simulink model "operator2"  (Simulink 8.1)
settings: Solver=ode45  StartTime=0.0  StopTime=inf  RelTol=1e-3
settings Model: Creator=eiseles  LastModifiedBy=eiseles
settings DataIOCC: SignalLoggingSaveFormat=Dataset
settings OptimizationCC: ExpressionDepthLimit=128
settings DebuggingCC: FcnCallInpInsideContextMsg=EnableAllAsError
settings GRTTargetCC: CombineOutputUpdateFcns=on  GRTInterface=off

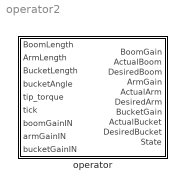
== system operator2 ==
  operator : Subsystem

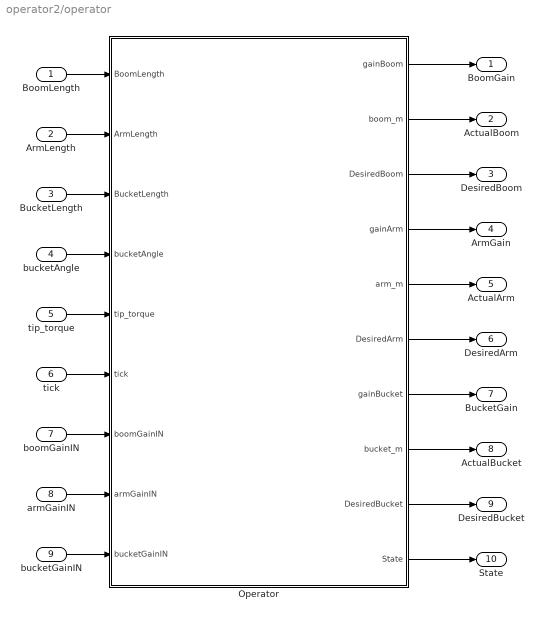
== system operator2/operator ==
  BoomLength : Inport
  ArmLength : Inport  Port=2
  BucketLength : Inport  Port=3
  bucketAngle : Inport  Port=4
  tip_torque : Inport  Port=5
  tick : Inport  Port=6
  boomGainIN : Inport  Port=7
  armGainIN : Inport  Port=8
  bucketGainIN : Inport  Port=9
  Operator : Stateflow chart  TreatAsAtomicUnit=on
  BoomGain : Outport
  ActualBoom : Outport  Port=2
  DesiredBoom : Outport  Port=3
  ArmGain : Outport  Port=4
  ActualArm : Outport  Port=5
  DesiredArm : Outport  Port=6
  BucketGain : Outport  Port=7
  ActualBucket : Outport  Port=8
  DesiredBucket : Outport  Port=9
  State : Outport  Port=10
  wires:
  bucketAngle/1 -> Operator/4(bucketAngle)
  BoomLength/1 -> Operator/1(BoomLength)
  BucketLength/1 -> Operator/3(BucketLength)
  tip_torque/1 -> Operator/5(tip_torque)
  ArmLength/1 -> Operator/2(ArmLength)
  Operator/2(boom_m) -> ActualBoom/1
  Operator/3(DesiredBoom) -> DesiredBoom/1
  Operator/4(gainArm) -> ArmGain/1
  Operator/1(gainBoom) -> BoomGain/1
  Operator/6(DesiredArm) -> DesiredArm/1
  Operator/7(gainBucket) -> BucketGain/1
  Operator/9(DesiredBucket) -> DesiredBucket/1
  Operator/5(arm_m) -> ActualArm/1
  Operator/8(bucket_m) -> ActualBucket/1
  tick/1 -> Operator/6(tick)
  Operator/10(State) -> State/1
  boomGainIN/1 -> Operator/7(boomGainIN)
  armGainIN/1 -> Operator/8(armGainIN)
  bucketGainIN/1 -> Operator/9(bucketGainIN)

== stateflow chart operator/Operator ==
  state captured
    entry: State= 1;
    boom_m = BoomLength;
    arm_m = ArmLength;
    bucket_m = -bucketAngle;
    DesiredBoom = .08;
    DesiredArm = .99;
    DesiredBucket = levelBucket;
    during:boom_m = BoomLength;
    arm_m = ArmLength;
    bucket_m = -bucketAngle;
  state Lifting
    entry: State= 2;
    boom_m = BoomLength;
    arm_m = ArmLength;
    bucket_m = -bucketAngle;
    DesiredBoom = .7;
    DesiredArm = .99;
    DesiredBucket = levelBucket;
    gainBoom = boomGainIN;
    gainArm = armGainIN;
    gainBucket = bucketGainIN;
    during:boom_m = BoomLength;
    arm_m = ArmLength;
    bucket_m = -bucketAngle;
  state Lifted
    entry: State= 3;
  state Extending
    entry: State= 4;
    boom_m = BoomLength;
    arm_m = ArmLength;
    bucket_m = -bucketAngle;
    DesiredBoom = .7;
    DesiredArm = .1;
    FinalArm = .1;
    DesiredBucket = levelBucket;
    gainArm = armGainIN*.3;
    during:boom_m = BoomLength;
    arm_m = ArmLength;
    bucket_m = -bucketAngle;
  state Extended
    entry: State= 6;
  state Dumping
    entry: State= 7;
    boom_m = BoomLength;
    arm_m = ArmLength;
    bucket_m = BucketLength;
    DesiredBoom = .7;
    DesiredArm = .1;
    DesiredBucket = .2;
    during: boom_m = BoomLength;
    arm_m = ArmLength;
    bucket_m = BucketLength;
  state Dumped
    en: State = 8;
    en,du: boom_m = BoomLength;
    arm_m = ArmLength;
    bucket_m = BucketLength;
  state bucketCyl_maxed
    entry: State = 5;
    DesiredBucket = .95;
    boom_m = BoomLength;
    arm_m = ArmLength;
    bucket_m = BucketLength;
    during:boom_m = BoomLength;
    arm_m = ArmLength;
    bucket_m = BucketLength;
  Extending -> bucketCyl_maxed [order 2] : [BucketLength>=.95]
  Lifted -> Extending : [tick==1]
  bucketCyl_maxed -> Dumping [order 2] : [-bucketAngle<=.6]
  bucketCyl_maxed -> Extended [order 1] : [arm_m<=FinalArm]
  Lifting -> Lifted : [boom_m>=DesiredBoom &&...
      |  arm_m >= DesiredArm]
  Extending -> Extended [order 1] : [arm_m<=FinalArm]
  Extended -> Dumping : [tick==1]
  captured -> Lifting : [tick==1]
  Dumping -> Dumped : [bucket_m<=DesiredBucket]
  (default) -> captured
  data: gainBoom output double =1; boom_m output double; DesiredBoom output double; gainArm output double =1; arm_m output double; DesiredArm output double; BoomLength input double; ArmLength input double; BucketLength input double; bucketAngle input double; gainBucket output double =1; bucket_m output double; DesiredBucket output double; tip_torque input double; max_torque local double =1e5; tick input double; State output double; FinalArm local double; levelBucket local double =1.8; boomGainIN input double; armGainIN input double; bucketGainIN input double
